simulink model "model4withDG"  (R2018b)
settings: Solver=VariableStepAuto  StartTime=0.0  StopTime=1  RelTol=1e-3
libraries: powerlib x25
settings Model: Creator=HP  LastModifiedBy=HP

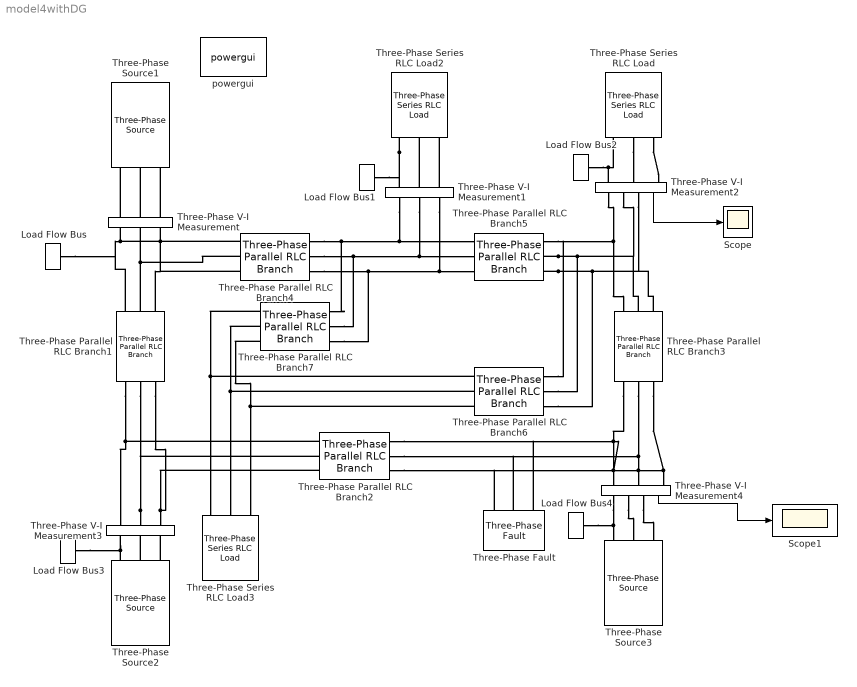
== system model4withDG ==
  Load Flow Bus : powerlib/Measurements/Load Flow Bus  LConnTagsString=a  Phases=single  Connectors=on one side  ID=BUS_1  Vbase=25e3  Vref=1.06  Vangle=0  VLF=1  VLFb=1  VLFc=1  angleLF=0  angleLFb=0  angleLFc=0
      settings: SourceProductName=Simscape Power Systems
  Load Flow Bus1 : powerlib/Measurements/Load Flow Bus  LConnTagsString=a  Phases=single  Connectors=on one side  ID=BUS_3  Vbase=25e3  Vref=1  Vangle=0  VLF=1  VLFb=1  VLFc=1  angleLF=0  angleLFb=0  angleLFc=0
      settings: SourceProductName=Simscape Power Systems
  Load Flow Bus2 : powerlib/Measurements/Load Flow Bus  LConnTagsString=a  Phases=single  Connectors=on one side  ID=BUS_4  Vbase=25e3  Vref=1  Vangle=0  VLF=1  VLFb=1  VLFc=1  angleLF=0  angleLFb=0  angleLFc=0
      settings: SourceProductName=Simscape Power Systems
  Load Flow Bus3 : powerlib/Measurements/Load Flow Bus  LConnTagsString=a  Phases=single  Connectors=on one side  ID=BUS_2  Vbase=25e3  Vref=1  Vangle=0  VLF=1  VLFb=1  VLFc=1  angleLF=0  angleLFb=0  angleLFc=0
      settings: SourceProductName=Simscape Power Systems
  Load Flow Bus4 : powerlib/Measurements/Load Flow Bus  LConnTagsString=a  Phases=single  Connectors=on one side  ID=BUS_5  Vbase=25e3  Vref=1  Vangle=0  VLF=1  VLFb=1  VLFc=1  angleLF=0  angleLFb=0  angleLFc=0
      settings: SourceProductName=Simscape Power Systems
  Scope : Scope
  Scope1 : Scope
  Three-Phase Parallel RLC Branch1 : powerlib/Elements/Three-Phase Parallel RLC Branch  LConnTagsString=A|B|C  RConnTagsString=A|B|C  BranchType=RL  Resistance=6  Inductance=1.9e-3  Capacitance=1e-6  Measurements=None
      settings: SourceProductName=Simscape Power Systems  SourceProductBaseCode=PS
  Three-Phase Parallel RLC Branch2 : powerlib/Elements/Three-Phase Parallel RLC Branch  LConnTagsString=A|B|C  RConnTagsString=A|B|C  BranchType=RL  Resistance=4  Inductance=3.8e-3  Capacitance=1e-6  Measurements=None
      settings: SourceProductName=Simscape Power Systems  SourceProductBaseCode=PS
  Three-Phase Parallel RLC Branch3 : powerlib/Elements/Three-Phase Parallel RLC Branch  LConnTagsString=A|B|C  RConnTagsString=A|B|C  BranchType=RL  Resistance=8  Inductance=7.63e-3  Capacitance=1e-6  Measurements=None
      settings: SourceProductName=Simscape Power Systems  SourceProductBaseCode=PS
  Three-Phase Parallel RLC Branch4 : powerlib/Elements/Three-Phase Parallel RLC Branch  LConnTagsString=A|B|C  RConnTagsString=A|B|C  BranchType=RL  Resistance=2  Inductance=7.63e-3  Capacitance=1e-6  Measurements=None
      settings: SourceProductName=Simscape Power Systems  SourceProductBaseCode=PS
  Three-Phase Parallel RLC Branch5 : powerlib/Elements/Three-Phase Parallel RLC Branch  LConnTagsString=A|B|C  RConnTagsString=A|B|C  BranchType=RL  Resistance=1  Inductance=0.95e-3  Capacitance=1e-6  Measurements=None
      settings: SourceProductName=Simscape Power Systems  SourceProductBaseCode=PS
  Three-Phase Parallel RLC Branch6 : powerlib/Elements/Three-Phase Parallel RLC Branch  LConnTagsString=A|B|C  RConnTagsString=A|B|C  BranchType=RL  Resistance=6  Inductance=5.7e-3  Capacitance=1e-6  Measurements=None
      settings: SourceProductName=Simscape Power Systems  SourceProductBaseCode=PS
  Three-Phase Parallel RLC Branch7 : powerlib/Elements/Three-Phase Parallel RLC Branch  LConnTagsString=A|B|C  RConnTagsString=A|B|C  BranchType=RL  Resistance=6  Inductance=5.7e-3  Capacitance=1e-6  Measurements=None
      settings: SourceProductName=Simscape Power Systems  SourceProductBaseCode=PS
  Three-Phase Series RLC Load : powerlib/Elements/Three-Phase Series RLC Load  LConnTagsString=A|B|C  Configuration=Y (grounded)  NominalVoltage=1000  Vabc=[1e3 1e3 1e3]  Vabcp=[1e3 1e3 1e3]  NominalFrequency=60  UnbalancedPower=off  ActivePower=40e6  InductivePower=5e6  CapacitivePower=0  Pabc=[10e3 9e3 11e3]  QLabc=[100 90 110]  QCabc=[100 90 110]  Pabcp=[10e3 9e3 11e3]  QLabcp=[100 90 110]  QCabcp=[100 90 110]  Measurements=None  LoadType=constant Z
  Three-Phase Series RLC Load2 : powerlib/Elements/Three-Phase Series RLC Load  LConnTagsString=A|B|C  Configuration=Y (grounded)  NominalVoltage=1000  Vabc=[1e3 1e3 1e3]  Vabcp=[1e3 1e3 1e3]  NominalFrequency=60  UnbalancedPower=off  ActivePower=45e6  InductivePower=15e6  CapacitivePower=0  Pabc=[10e3 9e3 11e3]  QLabc=[100 90 110]  QCabc=[100 90 110]  Pabcp=[10e3 9e3 11e3]  QLabcp=[100 90 110]  QCabcp=[100 90 110]  Measurements=None  LoadType=constant Z
  Three-Phase Series RLC Load3 : powerlib/Elements/Three-Phase Series RLC Load  LConnTagsString=A|B|C  Configuration=Y (grounded)  NominalVoltage=1000  Vabc=[1e3 1e3 1e3]  Vabcp=[1e3 1e3 1e3]  NominalFrequency=60  UnbalancedPower=off  ActivePower=20e6  InductivePower=10e6  CapacitivePower=0  Pabc=[10e3 9e3 11e3]  QLabc=[100 90 110]  QCabc=[100 90 110]  Pabcp=[10e3 9e3 11e3]  QLabcp=[100 90 110]  QCabcp=[100 90 110]  Measurements=None  LoadType=constant Z
  Three-Phase V-I Measurement : powerlib/Measurements/Three-Phase V-I Measurement  VoltageMeasurement=no  SetLabelV=off  LabelV=Vabc  Vpu=off  VpuLL=off  CurrentMeasurement=no  SetLabelI=off  LabelI=Iabc  Ipu=off  Pbase=100e6  Vbase=500e3  OutputType=Complex  PhasorSimulation=off  PSBequivalent=0
  Three-Phase V-I Measurement1 : powerlib/Measurements/Three-Phase V-I Measurement  VoltageMeasurement=no  SetLabelV=off  LabelV=Vabc  Vpu=off  VpuLL=off  CurrentMeasurement=no  SetLabelI=off  LabelI=Iabc  Ipu=off  Pbase=100e6  Vbase=500e3  OutputType=Complex  PhasorSimulation=off  PSBequivalent=0
  Three-Phase V-I Measurement2 : powerlib/Measurements/Three-Phase V-I Measurement  VoltageMeasurement=no  SetLabelV=off  LabelV=Vabc  Vpu=off  VpuLL=off  CurrentMeasurement=yes  SetLabelI=off  LabelI=Iabc  Ipu=off  Pbase=100e6  Vbase=500e3  OutputType=Complex  PhasorSimulation=off  PSBequivalent=0
  Three-Phase V-I Measurement3 : powerlib/Measurements/Three-Phase V-I Measurement  VoltageMeasurement=no  SetLabelV=off  LabelV=Vabc  Vpu=off  VpuLL=off  CurrentMeasurement=no  SetLabelI=off  LabelI=Iabc  Ipu=off  Pbase=100e6  Vbase=500e3  OutputType=Complex  PhasorSimulation=off  PSBequivalent=0
  Three-Phase V-I Measurement4 : powerlib/Measurements/Three-Phase V-I Measurement  VoltageMeasurement=no  SetLabelV=off  LabelV=Vabc  Vpu=off  VpuLL=off  CurrentMeasurement=yes  SetLabelI=off  LabelI=Iabc  Ipu=off  Pbase=100e6  Vbase=500e3  OutputType=Complex  PhasorSimulation=off  PSBequivalent=0
  Three-Phase Fault : powerlib/Elements/Three-Phase Fault  InitialStates=0  FaultA=on  FaultB=on  FaultC=on  GroundFault=on  SwitchTimes="[1/60  5/60]"  External=off  SwitchStatus=NaN  FaultResistance=0.001  GroundResistance=0.01  SnubberResistance=1e6  SnubberCapacitance=inf  Measurements=None
  Three-Phase Source1 : powerlib/Electrical Sources/Three-Phase Source  InternalConnection=Yg  VoltagePhases=off  Voltage=25e3  PhaseAngle=0  Voltage_phases=[25e3 25e3 25e3]/sqrt(3)  PhaseAngles_phases=[0 -120 +120]  Frequency=50  NonIdealSource=on  SpecifyImpedance=on  Resistance=0.8929  Inductance=16.58e-3  ShortCircuitLevel=100e6  BaseVoltage=25e3  XRratio=7  BusType=swing  Pref=10e3  Qref=0  Prefabc=[10e3, 10e3, 10e3]  Qrefabc=[0, 0, 0]  Qmin=-inf  Qmax=inf
  Three-Phase Source2 : powerlib/Electrical Sources/Three-Phase Source  InternalConnection=Yg  VoltagePhases=off  Voltage=25e3  PhaseAngle=0  Voltage_phases=[25e3 25e3 25e3]/sqrt(3)  PhaseAngles_phases=[0 -120 +120]  Frequency=50  NonIdealSource=on  SpecifyImpedance=on  Resistance=0.8929  Inductance=16.58e-3  ShortCircuitLevel=100e6  BaseVoltage=25e3  XRratio=7  BusType=swing  Pref=10e3  Qref=0  Prefabc=[10e3, 10e3, 10e3]  Qrefabc=[0, 0, 0]  Qmin=-inf  Qmax=inf
  Three-Phase Source3 : powerlib/Electrical Sources/Three-Phase Source  InternalConnection=Yg  VoltagePhases=off  Voltage=25e3  PhaseAngle=0  Voltage_phases=[25e3 25e3 25e3]/sqrt(3)  PhaseAngles_phases=[0 -120 +120]  Frequency=50  NonIdealSource=on  SpecifyImpedance=on  Resistance=0.8929  Inductance=16.58e-3  ShortCircuitLevel=100e6  BaseVoltage=25e3  XRratio=7  BusType=swing  Pref=10e3  Qref=0  Prefabc=[10e3, 10e3, 10e3]  Qrefabc=[0, 0, 0]  Qmin=-inf  Qmax=inf
  powergui : powerlib/powergui  Priority=1  SimulationMode=Continuous  SampleTime=50e-6  frequency=60  Iterations=50  frequencyindice=50  Pbase=100e6  ErrMax=1e-4  UnitsV=kV  UnitsW=MW  buscounter=0  FunctionMessages=off  echomessages=off  EnableUseOfTLC=off  CurrentSourceSwitches=off  DisableSnubberDevices=off  DisableRonSwitches=off  DisableVfSwitches=off  DisplayEquations=off  SolverType=Tustin/Backward Euler (TBE)  Interpol=off  ExternalGateDelay=off  methode=off  Ts=100  x0status=blocks  SPID=off  SwTol=0  HookPort=off  RestoreLinks=warning  ResistiveCurrentMeasurement=off  Frange=[0:2:500]  Ylog=off  Xlog=on  ShowGrid=off  save=off  variable=ZData  structure=0  ZoomFFT=off  StartTime=0.0  cycles=1  DisplayStyle=1  fundamental=60  FreqAxis=off  MaxFrequency=1000  frequencyindicesteady=1  RmsSteady=1  display=off
  wires:
  Three-Phase V-I Measurement2/1 -> Scope/1
  Three-Phase V-I Measurement4/1 -> Scope1/1
  connections:
  Three-Phase V-I Measurement4/LConn2 -- Three-Phase Fault/LConn2 -- Three-Phase Parallel RLC Branch2/RConn2 -- Three-Phase Parallel RLC Branch3/RConn2
  Three-Phase V-I Measurement2/LConn3 -- Three-Phase Series RLC Load/LConn1 -- Load Flow Bus2/LConn1
  Three-Phase Parallel RLC Branch5/RConn3 -- Three-Phase Parallel RLC Branch6/RConn3 -- Three-Phase Parallel RLC Branch3/LConn3 -- Three-Phase V-I Measurement2/RConn1
  Three-Phase Parallel RLC Branch4/RConn2 -- Three-Phase Parallel RLC Branch7/RConn2 -- Three-Phase Parallel RLC Branch5/LConn2 -- Three-Phase V-I Measurement1/RConn2
  Three-Phase Parallel RLC Branch7/LConn2 -- Three-Phase Parallel RLC Branch6/LConn2 -- Three-Phase Series RLC Load3/LConn2
  Three-Phase Parallel RLC Branch1/RConn1 -- Three-Phase Parallel RLC Branch2/LConn1 -- Three-Phase V-I Measurement3/LConn3
  Three-Phase V-I Measurement/RConn3 -- Three-Phase Parallel RLC Branch4/LConn1 -- Load Flow Bus/LConn1 -- Three-Phase Parallel RLC Branch1/LConn1
  Three-Phase Parallel RLC Branch4/RConn3 -- Three-Phase Parallel RLC Branch7/RConn3 -- Three-Phase Parallel RLC Branch5/LConn3 -- Three-Phase V-I Measurement1/RConn1
  Three-Phase Parallel RLC Branch1/LConn2 -- Three-Phase V-I Measurement/RConn2 -- Three-Phase Parallel RLC Branch4/LConn2
  Three-Phase Parallel RLC Branch5/RConn2 -- Three-Phase Parallel RLC Branch6/RConn2 -- Three-Phase Parallel RLC Branch3/LConn2 -- Three-Phase V-I Measurement2/RConn2
  Three-Phase V-I Measurement3/RConn3 -- Three-Phase Source2/RConn1 -- Load Flow Bus3/LConn1
  Three-Phase V-I Measurement3/LConn2 -- Three-Phase Parallel RLC Branch2/LConn2 -- Three-Phase Parallel RLC Branch1/RConn2
  Three-Phase V-I Measurement4/LConn1 -- Three-Phase Parallel RLC Branch3/RConn3 -- Three-Phase Fault/LConn3 -- Three-Phase Parallel RLC Branch2/RConn3
  Three-Phase V-I Measurement2/RConn3 -- Three-Phase Parallel RLC Branch6/RConn1 -- Three-Phase Parallel RLC Branch5/RConn1 -- Three-Phase Parallel RLC Branch3/LConn1
  Three-Phase V-I Measurement/RConn1 -- Three-Phase Parallel RLC Branch1/LConn3 -- Three-Phase Parallel RLC Branch4/LConn3
  Three-Phase Series RLC Load2/LConn1 -- Load Flow Bus1/LConn1 -- Three-Phase V-I Measurement1/LConn3
  Three-Phase V-I Measurement4/LConn3 -- Three-Phase Fault/LConn1 -- Three-Phase Parallel RLC Branch2/RConn1 -- Three-Phase Parallel RLC Branch3/RConn1
  Three-Phase Parallel RLC Branch7/LConn3 -- Three-Phase Parallel RLC Branch6/LConn3 -- Three-Phase Series RLC Load3/LConn3
  Three-Phase V-I Measurement3/LConn1 -- Three-Phase Parallel RLC Branch2/LConn3 -- Three-Phase Parallel RLC Branch1/RConn3
  Three-Phase Parallel RLC Branch4/RConn1 -- Three-Phase Parallel RLC Branch7/RConn1 -- Three-Phase V-I Measurement1/RConn3 -- Three-Phase Parallel RLC Branch5/LConn1
  Three-Phase Parallel RLC Branch7/LConn1 -- Three-Phase Parallel RLC Branch6/LConn1 -- Three-Phase Series RLC Load3/LConn1
  Three-Phase V-I Measurement/LConn2 -- Three-Phase Source1/RConn2
  Three-Phase V-I Measurement/LConn1 -- Three-Phase Source1/RConn3
  Three-Phase Source2/RConn3 -- Three-Phase V-I Measurement3/RConn1
  Three-Phase Series RLC Load/LConn3 -- Three-Phase V-I Measurement2/LConn1
  Three-Phase V-I Measurement/LConn3 -- Three-Phase Source1/RConn1
  Three-Phase V-I Measurement1/LConn1 -- Three-Phase Series RLC Load2/LConn3
  Three-Phase V-I Measurement1/LConn2 -- Three-Phase Series RLC Load2/LConn2
  Three-Phase Series RLC Load/LConn2 -- Three-Phase V-I Measurement2/LConn2
  Three-Phase Source2/RConn2 -- Three-Phase V-I Measurement3/RConn2
  Three-Phase V-I Measurement4/RConn3 -- Load Flow Bus4/LConn1 -- Three-Phase Source3/RConn3
  Three-Phase V-I Measurement4/RConn2 -- Three-Phase Source3/RConn2
  Three-Phase V-I Measurement4/RConn1 -- Three-Phase Source3/RConn1
